simulink model "integrated2"  (R2021b)
settings: Solver=VariableStepAuto  StartTime=0.0  StopTime=10.0  RelTol=1e-3
values from neighbouring files (symbols this model uses):
  C = [1, 0, 0, 0, 0, 0 ... (first row only)    [integrated.m]    (also in parse3e4_kalmanComBias.m = [1 0]; parse3e4_kalmanSemBias.m = 1)
  Q = [0.05, 0, 0, 0, 0, 0 ... (first row only)    [integrated.m]
  R = [0.05, 0, 0 ... (first row only)    [integrated.m]
  sampleTime = 0.005    [sensorsA.mat]    (also in sensorsB2.mat; sensorsC.mat)
settings Model: Creator=arthurlago  LastModifiedBy=arthurlago

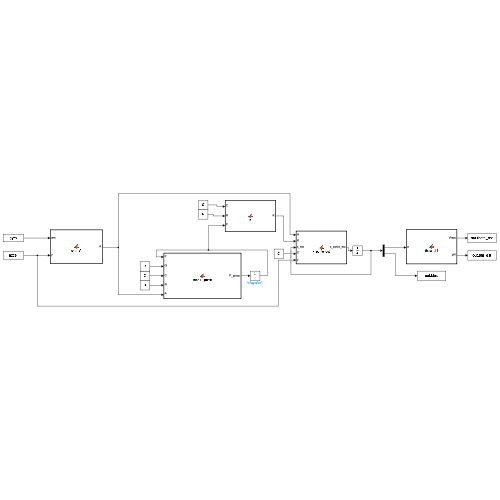
[thumbnail: Simulink's stored preview of the top-level diagram]
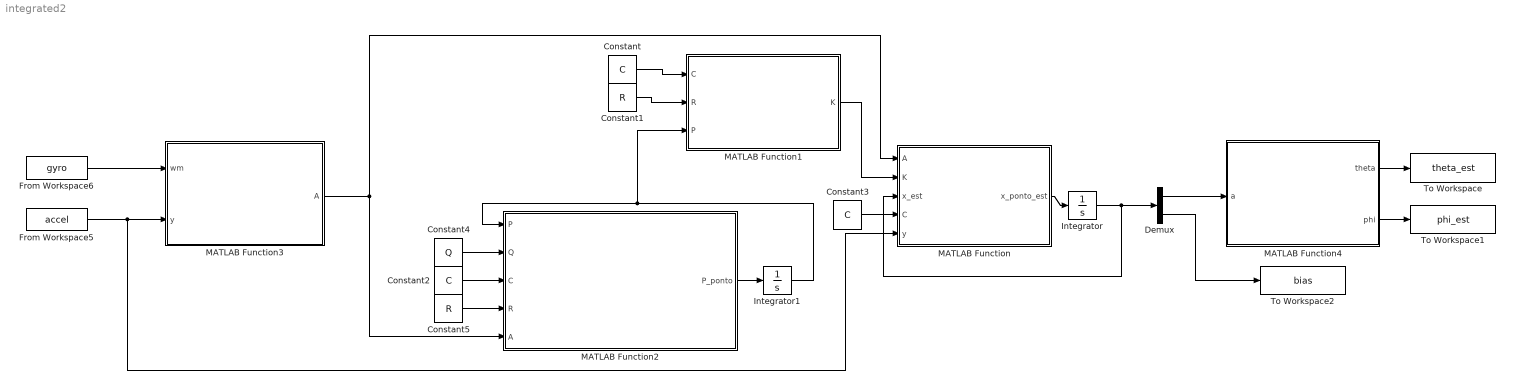
== system integrated2 ==
  Constant : Constant  Value=C  SampleTime=sampleTime
  Constant1 : Constant  Value=R  SampleTime=sampleTime
  Constant2 : Constant  Value=C  SampleTime=sampleTime
  Constant3 : Constant  Value=C  SampleTime=sampleTime
  Constant4 : Constant  Value=Q  SampleTime=sampleTime
  Constant5 : Constant  Value=R  SampleTime=sampleTime
  Demux : Demux  Outputs=2
  From Workspace5 : FromWorkspace  VariableName=accel  SampleTime=sampleTime
  From Workspace6 : FromWorkspace  VariableName=gyro  SampleTime=sampleTime
  Integrator : Integrator
  Integrator1 : Integrator
  MATLAB Function : MATLAB Function  TreatAsAtomicUnit=on
  MATLAB Function1 : MATLAB Function  TreatAsAtomicUnit=on
  MATLAB Function2 : MATLAB Function  TreatAsAtomicUnit=on
  MATLAB Function3 : MATLAB Function  TreatAsAtomicUnit=on
  MATLAB Function4 : MATLAB Function  TreatAsAtomicUnit=on
  To Workspace : ToWorkspace  VariableName=theta_est  SaveFormat=Timeseries  SampleTime=-1
  To Workspace1 : ToWorkspace  VariableName=phi_est  SaveFormat=Timeseries  SampleTime=-1
  To Workspace2 : ToWorkspace  VariableName=bias  SaveFormat=Timeseries  SampleTime=-1
  wires:
  MATLAB Function/1(x_ponto_est) -> Integrator/1
  Integrator/1 -> Demux/1, MATLAB Function/3(x_est)
  MATLAB Function1/1(K) -> MATLAB Function/2(K)
  Constant1/1 -> MATLAB Function1/2(R)
  Constant/1 -> MATLAB Function1/1(C)
  Constant5/1 -> MATLAB Function2/4(R)
  Constant2/1 -> MATLAB Function2/3(C)
  Constant4/1 -> MATLAB Function2/2(Q)
  MATLAB Function3/1(A) -> MATLAB Function/1(A), MATLAB Function2/5(A)
  From Workspace5/1 -> MATLAB Function/5(y), MATLAB Function3/2(y)
  From Workspace6/1 -> MATLAB Function3/1(wm)
  Demux/1 -> MATLAB Function4/1(a)
  MATLAB Function4/1(theta) -> To Workspace/1
  MATLAB Function4/2(phi) -> To Workspace1/1
  Demux/2 -> To Workspace2/1
  Constant3/1 -> MATLAB Function/4(C)
  MATLAB Function2/1(P_ponto) -> Integrator1/1
  Integrator1/1 -> MATLAB Function1/3(P), MATLAB Function2/1(P)

== matlab function integrated2/MATLAB Function1 ==
  data: C input; K output; R input; P input
function K = K(C, R, P)
    CT = transpose(C);
    Rinv = inv(R);
    K = P*CT*Rinv;
end

== matlab function integrated2/MATLAB Function ==
  data: A input; x_ponto_est output; K input; x_est input; C input; y input
function x_ponto_est = x_ponto_est(A, K, x_est, C, y)
    x_ponto_est=[0;0;0;0;0;0];
    res = y - C*x_est;
    x_ponto_est =A*x_est+K*res ;
end

== matlab function integrated2/MATLAB Function2 ==
  data: P input; P_ponto output; Q input; C input; R input; A input
function P_ponto =criar_P_ponto(P, Q, C, R, A)
    AT = transpose(A);
    CT = transpose(C);
    Rinv = inv(R);
    P_ponto = A*P + P*AT + Q - P*CT*Rinv*C*P;
end

== matlab function integrated2/MATLAB Function3 ==
  data: wm input; A output; y input
function A =criar_A(wm, y)
    w_x = wm(1);
    w_y = wm(2);
    w_z = wm(3);
    
    y_ax = y(1);
    y_ay = y(2);
    y_az = y(3);
    
    A = [0 w_z -w_y 0 y_az -y_ay;
         -w_z 0 w_x -y_az 0 y_ax;
         w_y -w_x 0 y_ay -y_ax 0;
         0 0 0 0 0 0;
         0 0 0 0 0 0;
         0 0 0 0 0 0];

end

== matlab function integrated2/MATLAB Function4 ==
  data: a input; theta output; phi output
function [theta, phi] = theta_phi(a)
    phi = 180/pi*atan(a(2)/ a(3));
    theta = 180/pi*atan(a(1)/sqrt(a(2)^2 + a(3)^2));
end
